simulink model "Que3_4"  (R2023b)
settings: Solver=VariableStepAuto  StartTime=0.0  StopTime=100.0  MaxStep=75e-6  RelTol=1e-3
settings Model: Creator=setak  LastModifiedBy=setak

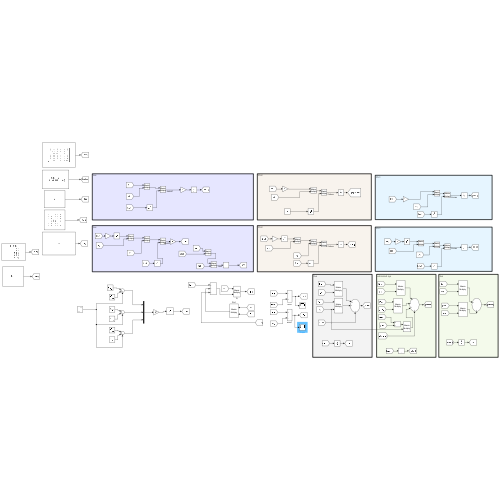
[thumbnail: Simulink's stored preview of the top-level diagram]
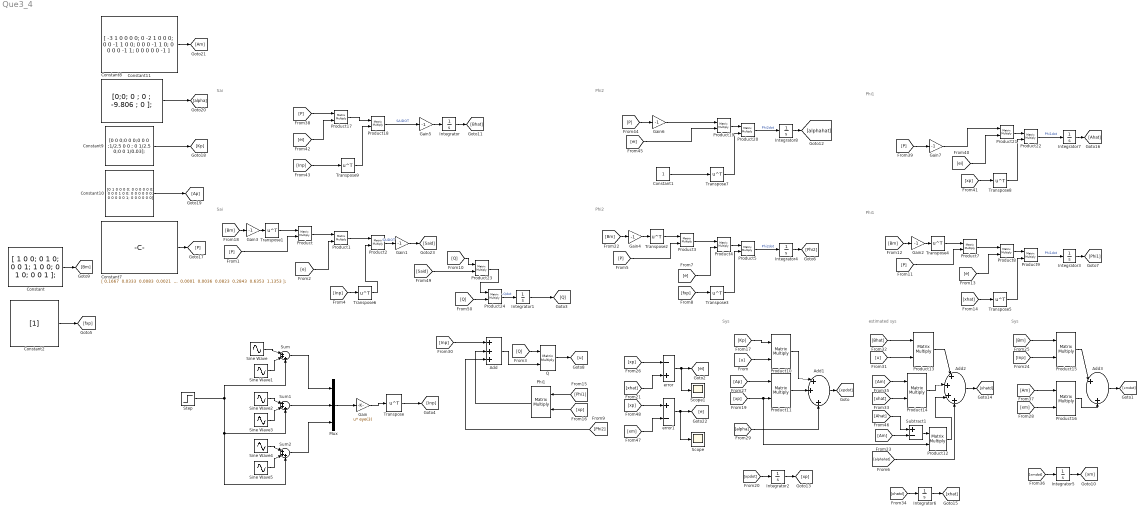
== system Que3_4 ==
  note: Phi1
  note: Sai
  note: Phi2
  note: Sys
  note: estimated sys
  note: Sys
  note: Phi1
  note: Phi2
  note: Sai
  Add : Sum  Inputs=+++
  Add1 : Sum  Inputs=|++|+
  Add2 : Sum  Inputs=|+|+|+|+
  Add3 : Sum  Inputs=|+|+
  Constant : Constant  Value=|
      | [ 1 0 0;
      |            0 1 0;
      |            0 0 1;
      |            1 0 0;
      |            0 1 0;
      |            0 0 1 ];
  Constant1 : Constant
  Constant10 : Constant  Value=|
      | [0 1 0 0 0 0;      0 0 0 0 0 0;
      |       0 0 0 1 0 0;      0 0 0 0 0 0;
      |       0 0 0 0 0 1;      0 0 0 0 0 0]
  Constant11 : Constant  Value=|
      | [ -3  1  0  0  0  0;
      |             0 -2  1  0  0  0;
      |             0  0 -1  1  0  0;
      |             0  0  0 -1  1  0;
      |             0  0  0  0 -1  1;
      |             0  0  0  0  0 -1 ]
  Constant2 : Constant  Value=[1]
  Constant7 : Constant  Value=|
      | [ 0.1667  0.0333  0.0083  0.0021  0.0005  0.0001;
      |           0.0333  0.2667  0.0917  0.0312  0.0106  0.0036;
      |           0.0083  0.0917  0.5917  0.3115  0.1610  0.0823;
      |           0.0021  0.0312  0.3115  0.8115  0.4862  0.2843;
      |           0.0005  0.0106  0.1610  0.4862  0.9862  0.6353;
      |           0.0001  0.0036  0.0823  0.2843  0.6353  1.1353 ];
  Constant8 : Constant  Value=|
      | [0;0;      0 ;
      |       0 ;  -9.806 ;      0 ];
  Constant9 : Constant  Value="[0 0 0;0 0 0;0 0 0 ;1/2.5 0 0  ; 0 1/2.5  0;0 0 1/0.03];"
  Gain : Gain  Gain=eye(3)  Multiplication=Matrix(u*K)
  Gain{1..7} (7 alike) : Gain  Gain=-1
  Integrator{,3..4,7..8} (5 alike) : Integrator
  Integrator1 : Integrator  InitialCondition=[0 0 0; 0 0 0; 0 0 0]  IgnoreLimit=on
  Integrator2 : Integrator  InitialCondition=[0 ;0; 0;0;0;0]
  Integrator5 : Integrator  InitialCondition=[0.01;0.01;0.01;0.01;0.01;0.01;]
  Integrator6 : Integrator  InitialCondition=[0; 0; 0;0;0;0]
  Mux : Mux  Inputs=3
  Phi1 : Product  Multiplication=Matrix(*)
  Product{,1..5,7..24} (24 alike) : Product  Multiplication=Matrix(*)
  Q : Product  Multiplication=Matrix(*)
  Scope : Scope
  Scope1 : Scope
  Sine Wave : Sin  Frequency=2  SampleTime=0
  Sine Wave1 : Sin  Amplitude=3  Frequency=4  SampleTime=0
  Sine Wave2 : Sin  Amplitude=2  Frequency=4  SampleTime=0
  Sine Wave3 : Sin  Amplitude=3  Frequency=6  SampleTime=0
  Sine Wave4 : Sin  Amplitude=3  Frequency=9  SampleTime=0
  Sine Wave5 : Sin  Amplitude=4  Frequency=12  SampleTime=0
  Step : Step  Before=2  After=3  SampleTime=0
  Subtract1 : Sum  Inputs=+-
  Sum : Sum  Inputs=|+++
  Sum1 : Sum  Inputs=|+++
  Sum2 : Sum  Inputs=|+++
  Transpose{,1..9} (10 alike) : Math  Operator=transpose
  error : Sum  Inputs=-+
  error1 : Sum  Inputs=+-
  wires:
  Constant7/1 -> [P]
  Constant11/1 -> [Am]
  Constant10/1 -> [Ap]
  Constant8/1 -> [alpha]
  Gain3/1 -> Transpose1/1
  Gain4/1 -> Transpose2/1
  Gain2/1 -> Transpose4/1
  [Q] -> Product23/1
  [Bm] -> Gain4/1
  Transpose4/1 -> Product7/1
  Transpose6/1 -> Product2/2
  Product3/1 -> Product4/1
  [xhat] -> error/2
  [xp] -> error/1
  Integrator4/1 -> [Phi2]
  [Inp] -> Transpose6/1
  Constant2/1 -> [fxp]
  [xp] -> Phi1/2
  Sine Wave5/1 -> Sum2/2
  [Phi1] -> Phi1/1
  [fxp] -> Transpose3/1
  Gain/1 -> Transpose/1
  Product4/1 -> Product5/1
  Constant9/1 -> [Kp]
  Transpose3/1 -> Product5/2
  [xhat] -> Transpose5/1
  Product5/1 -> Integrator4/1  "Phi2dot"
  Constant/1 -> [Bm]
  Product8/1 -> Product9/1
  Product1/1 -> Product2/1
  Product7/1 -> Product8/1
  Transpose5/1 -> Product9/2
  [P] -> Product7/2
  [e] -> Product4/2
  Add/1 -> Q/2
  Product2/1 -> Gain1/1  "SAIDOT"
  Product9/1 -> Integrator3/1  "Phi1dot"
  Transpose1/1 -> Product/1
  error/1 -> Scope1/1, [ei]
  [e] -> Product1/2
  [Inp] -> Add/1
  Transpose2/1 -> Product3/1
  Product/1 -> Product1/1
  [Q] -> Q/1
  Step/1 -> Sum2/3, Sum1/3, Sum/3
  [P] -> Product3/2
  [Bm] -> Gain2/1
  Integrator1/1 -> [Q]
  [Bm] -> Gain3/1
  Sum/1 -> Mux/1
  [e] -> Product8/2
  Sum2/1 -> Mux/3
  Sine Wave1/1 -> Sum/2
  Transpose/1 -> [Inp]
  Sine Wave2/1 -> Sum1/1
  Sum1/1 -> Mux/2
  [P] -> Product/2
  Sine Wave4/1 -> Sum2/1
  Sine Wave/1 -> Sum/1
  [Phi2] -> Add/3
  Phi1/1 -> Add/2
  Integrator3/1 -> [Phi1]
  Sine Wave3/1 -> Sum1/2
  Q/1 -> [u]
  Mux/1 -> Gain/1
  Add1/1 -> [xpdot]
  [alpha] -> Add1/3
  [Bhat] -> Product13/1
  Integrator2/1 -> [xp]
  [Ap] -> Product11/1
  [u] -> Product10/2
  [xp] -> Product12/2, Product11/2
  [Am] -> Product14/1
  Product14/1 -> Add2/2
  Add2/1 -> [xhatd]
  Subtract1/1 -> Product12/1
  [xpdot] -> Integrator2/1
  Product12/1 -> Add2/3
  [Am] -> Subtract1/2
  Product13/1 -> Add2/1
  [alphahat] -> Add2/4
  Product11/1 -> Add1/2
  Integrator6/1 -> [xhat]
  [xhat] -> Product14/2
  [xhatd] -> Integrator6/1
  [Kp] -> Product10/1
  Product10/1 -> Add1/1
  [u] -> Product13/2
  [Bm] -> Product15/1
  Add3/1 -> [xmdot]
  Integrator5/1 -> [xm]
  [xmdot] -> Integrator5/1
  Product15/1 -> Add3/1
  [Inp] -> Product15/2
  [xm] -> Product16/2
  Product16/1 -> Add3/2
  [Am] -> Product16/1
  Constant1/1 -> Transpose7/1
  Product18/1 -> Gain5/1  "SAIDOT"
  Transpose9/1 -> Product18/2
  [Inp] -> Transpose9/1
  [P] -> Gain6/1
  Product17/1 -> Product18/1
  [P] -> Product17/1
  [P] -> Gain7/1
  Gain7/1 -> Product21/1
  Product22/1 -> Integrator7/1  "Phi1dot"
  Product19/1 -> Product20/1
  [ei] -> Product19/2
  Integrator/1 -> [Bhat]
  Gain5/1 -> Integrator/1
  [ei] -> Product17/2
  Gain6/1 -> Product19/1
  Transpose7/1 -> Product20/2
  Product21/1 -> Product22/1
  Transpose8/1 -> Product22/2
  Integrator7/1 -> [Ahat]
  Integrator8/1 -> [alphahat]
  Product20/1 -> Integrator8/1  "Phi2dot"
  [ei] -> Product21/2
  [Ahat] -> Subtract1/1
  [xp] -> error1/1
  [xm] -> error1/2
  [xp] -> Transpose8/1
  Product24/1 -> Integrator1/1  "-Qdot"
  Gain1/1 -> [Said]
  [Said] -> Product23/2
  Product23/1 -> Product24/1
  [Q] -> Product24/2
  error1/1 -> Scope/1, [e]
